simulink model "InvPendulum"  (R2021b)
settings: Solver=VariableStepAuto  StartTime=0.0  StopTime=10.0  RelTol=1e-3
undefined symbols (not defined in the file or in its folder): drawPendulum
libraries: simulink x2
settings Model: Creator=zhour  LastModifiedBy=zhour

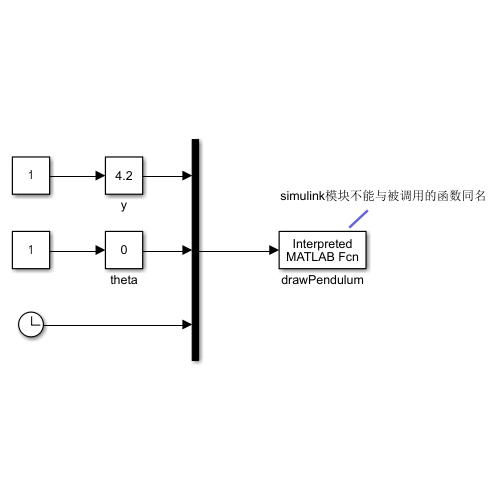
[thumbnail: Simulink's stored preview of the top-level diagram]
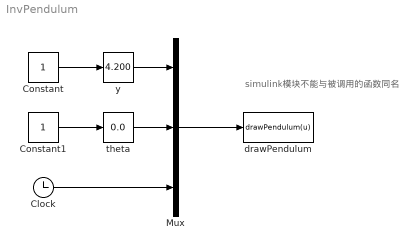
== system InvPendulum ==
  note: simulink模块不能与被调用的函数同名
  Clock : Clock
  Constant : Constant
  Constant1 : Constant
  Mux : Mux  Inputs=3
  drawPendulum : MATLABFcn  MATLABFcn=drawPendulum(u)  OutputDimensions=0
  theta : simulink/Math Operations/Slider Gain  gain=0.0  low=-30  high=30
  y : simulink/Math Operations/Slider Gain  gain=4.200  low=-10  high=10
  wires:
  Constant/1 -> y/1
  Constant1/1 -> theta/1
  y/1 -> Mux/1
  theta/1 -> Mux/2
  Clock/1 -> Mux/3
  Mux/1 -> drawPendulum/1
